simulink model "SimulinkTCPA_trial2"  (R2020a)
settings: Solver=VariableStepAuto  StartTime=0.0  StopTime=10.0  RelTol=1e-3
settings Model: Creator=manth  LastModifiedBy=manth

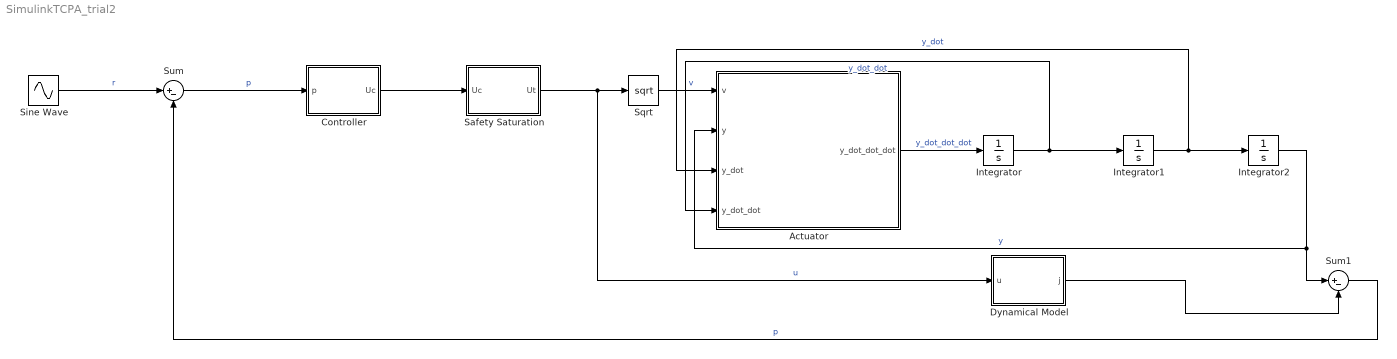
== system SimulinkTCPA_trial2 ==
  Actuator : MATLAB Function  TreatAsAtomicUnit=on
  Controller : MATLAB Function  TreatAsAtomicUnit=on
  Dynamical Model : MATLAB Function  TreatAsAtomicUnit=on
  Integrator : Integrator
  Integrator1 : Integrator
  Integrator2 : Integrator
  Safety Saturation : MATLAB Function  TreatAsAtomicUnit=on
  Sine Wave : Sin  Amplitude=2  Frequency=0.62831853  SampleTime=0
  Sqrt : Sqrt  SaturateOnIntegerOverflow=on
  Sum : Sum  Inputs=|+-
  Sum1 : Sum  Inputs=|+-
  wires:
  Sine Wave/1 -> Sum/1  "r"
  Sum/1 -> Controller/1(p)  "p"
  Controller/1(Uc) -> Safety Saturation/1(Uc)
  Safety Saturation/1(Ut) -> Dynamical Model/1(u), Sqrt/1  "u"
  Sqrt/1 -> Actuator/1(v)  "v"
  Actuator/1(y_dot_dot_dot) -> Integrator/1  "y_dot_dot_dot"
  Integrator/1 -> Actuator/4(y_dot_dot), Integrator1/1  "y_dot_dot"
  Integrator1/1 -> Actuator/3(y_dot), Integrator2/1  "y_dot"
  Integrator2/1 -> Actuator/2(y), Sum1/1  "y"
  Dynamical Model/1(j) -> Sum1/2
  Sum1/1 -> Sum/2  "p"

== matlab function SimulinkTCPA_trial2/Safety Saturation ==
  data: Uc input; Ut output
function Ut = Saturation(Uc)



if (100<Uc)
    Ut=100;
    
elseif (Uc<0)
    Ut=0;
else 
    Ut=Uc;
end

== matlab function SimulinkTCPA_trial2/Controller ==
  data: p input; Uc output
function Uc = Gc(p)

L=0.5;
b0=42.09;
a0=44.09;
a1=1003;
a2=371.1;


F=  tf([1],[L^3 3*L^2 3*L 1]);
Gd= tf([b0],[1 a2 a1 a0]);

Gc=F/Gd;

Uc=Gc*(p);

== matlab function SimulinkTCPA_trial2/Actuator ==
  data: v input; y input; y_dot_dot_dot output; y_dot input; y_dot_dot input
function y_dot_dot_dot = TCPA_Actuator(v,y,y_dot,y_dot_dot)

b0=42.09;
a0=44.09;
a1=1003;
a2=371.1;

y_dot_dot_dot = (b0*(v^2)) - (a2*y_dot_dot) - (a1*y_dot) - (a0*y);

== matlab function SimulinkTCPA_trial2/Dynamical Model ==
  data: u input; j output
function j = GD(u)


b0=42.09;
a0=44.09;
a1=1003;
a2=371.1;

Gd= tf([b0],[1 a2 a1 a0]);

j=Gd*u;
